simulink model "controller_2013B"  (R2013b)
settings: Solver=ode45  StartTime=0.0  StopTime=sim_time  FixedStep=0.001  RelTol=1e-3
InitFcn:
  | zh = 0.01;
undefined symbols (not defined in the file): Standard_Devices, UDP_Protocol, zh_step
libraries: rtwinlib x6, simulink x2, commutil2 x2, dspnetwork x2
settings Model: Creator=Lenka  LastModifiedBy=Anony
settings DebuggingCC: UnderspecifiedInitializationDetection=Simplified  MergeDetectMultiDrivingBlocksExec=error  FrameProcessingCompatibilityMsg=error
settings GRTTargetCC: CodeReplacementLibrary=C89/C90 (ANSI)

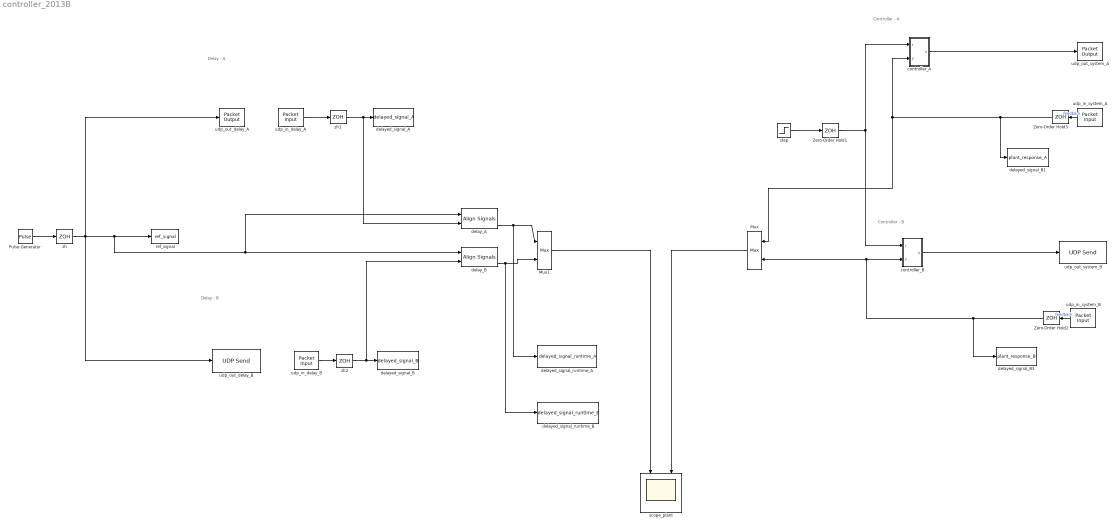
== system controller_2013B ==
  note: Controller - B
  note: Controller - A
  note: Delay - A
  note: Delay - B
  Mux : Mux  Inputs=2
  Mux1 : Mux  Inputs=2
  Pulse Generator : DiscretePulseGenerator  PulseType=Time based  Period=0.5  PulseWidth=0.1
  Zero-Order Hold1 : ZeroOrderHold  SampleTime=zh_step
  Zero-Order Hold2 : ZeroOrderHold  SampleTime=zh_step
  Zero-Order Hold3 : ZeroOrderHold  SampleTime=zh_step
  controller_A : Subsystem
  controller_B : Subsystem
  delay_A : commutil2/Align Signals  corrLength=800  stopUpdate=off  numConstDelay=3
  delay_B : commutil2/Align Signals  corrLength=800  stopUpdate=off  numConstDelay=3
  delayed_signal_A : ToWorkspace  VariableName=delayed_signal_A  SampleTime=zh_step  SaveFormat=Timeseries
  delayed_signal_B : ToWorkspace  VariableName=delayed_signal_B  SampleTime=zh_step  SaveFormat=Timeseries
  delayed_signal_B1 : ToWorkspace  VariableName=plant_response_A  SampleTime=zh_step  SaveFormat=Timeseries
  delayed_signal_B3 : ToWorkspace  VariableName=plant_response_B  SampleTime=zh_step  SaveFormat=Timeseries
  delayed_signal_runtime_A : ToWorkspace  VariableName=delayed_signal_runtime_A  SampleTime=zh_step  SaveFormat=Timeseries
  delayed_signal_runtime_B : ToWorkspace  VariableName=delayed_signal_runtime_B  SampleTime=zh_step  SaveFormat=Timeseries
  ref_signal : ToWorkspace  VariableName=ref_signal  SampleTime=zh_step  SaveFormat=Timeseries
  scope_plant : Scope  NumInputPorts=2
      settings: ShowLegends=on  YMin=0~0  YMax=325~1.3
  step : Step  SampleTime=0
  udp_in_delay_A : rtwinlib/Packet Input  SampleTime=0.001  MaxMissedTicks=inf  ShowMissedTicks=off  YieldWhenWaiting=off  DrvName=Standard_Devices/UDP_Protocol  DrvAddress=28000  DrvOptions=[2468394757 28000]  PacketSize=8  DataTypes='double'  ShowReady=off  ShowError=off  PacketID=1  ByteOrder=1  ShowTimestamp=off
      settings: AttributesFormatString=Standard Devices\nUDP Protocol [6978h]
  udp_in_delay_B : rtwinlib/Packet Input  SampleTime=0.001  MaxMissedTicks=inf  ShowMissedTicks=off  YieldWhenWaiting=off  DrvName=Standard_Devices/UDP_Protocol  DrvAddress=28010  DrvOptions=[2468394757 28010]  PacketSize=8  DataTypes='double'  ShowReady=off  ShowError=off  PacketID=1  ByteOrder=1  ShowTimestamp=off
      settings: AttributesFormatString=Standard Devices\nUDP Protocol [6982h]
  udp_in_system_A : rtwinlib/Packet Input  SampleTime=0.001  MaxMissedTicks=inf  ShowMissedTicks=off  YieldWhenWaiting=off  DrvName=Standard_Devices/UDP_Protocol  DrvAddress=28500  DrvOptions=[2468394757 28500]  PacketSize=8  DataTypes='double'  ShowReady=off  ShowError=off  PacketID=1  ByteOrder=1  ShowTimestamp=off
      settings: AttributesFormatString=Standard Devices\nUDP Protocol [6F54h]
  udp_in_system_B : rtwinlib/Packet Input  SampleTime=0.001  MaxMissedTicks=inf  ShowMissedTicks=off  YieldWhenWaiting=off  DrvName=Standard_Devices/UDP_Protocol  DrvAddress=28510  DrvOptions=[2468394757 28510]  PacketSize=8  DataTypes='double'  ShowReady=off  ShowError=off  PacketID=1  ByteOrder=1  ShowTimestamp=off
      settings: AttributesFormatString=Standard Devices\nUDP Protocol [6F54h]
  udp_out_delay_A : rtwinlib/Packet Output  SampleTime=0.01  MaxMissedTicks=inf  ShowMissedTicks=off  YieldWhenWaiting=off  DrvName=Standard_Devices/UDP_Protocol  DrvAddress=27000  DrvOptions=[2468394757 27000]  PacketSize=8  DataTypes='double'  ShowReady=off  ShowError=off  PacketID=1  ByteOrder=1  InitialValue=[]  FinalValue=[]
      settings: AttributesFormatString=Standard Devices\nUDP Protocol [6D60h]
  udp_out_delay_B : dspnetwork/UDP Send  remoteURL='147.32.183.5'  remotePort=27010  localURL='0.0.0.0'  localPortSource=Automatically determine  localPort=27000  sampletime=-1  separateLengthPort=0
  udp_out_system_A : rtwinlib/Packet Output  SampleTime=0.01  MaxMissedTicks=inf  ShowMissedTicks=off  YieldWhenWaiting=off  DrvName=Standard_Devices/UDP_Protocol  DrvAddress=27500  DrvOptions=[2468394757 27500]  PacketSize=8  DataTypes='double'  ShowReady=off  ShowError=off  PacketID=1  ByteOrder=1  InitialValue=[]  FinalValue=[]
      settings: AttributesFormatString=Standard Devices\nUDP Protocol [6B6Ch]
  udp_out_system_B : dspnetwork/UDP Send  remoteURL='147.32.183.5'  remotePort=27510  localURL='0.0.0.0'  localPortSource=Automatically determine  localPort=27000  sampletime=-1  separateLengthPort=0
  zh : ZeroOrderHold  SampleTime=zh_step
  zh1 : ZeroOrderHold  SampleTime=zh_step
  zh2 : ZeroOrderHold  SampleTime=zh_step
  wires:
  udp_in_system_A/1 -> Zero-Order Hold3/1  "feedback"
  step/1 -> Zero-Order Hold1/1
  controller_A/1(u) -> udp_out_system_A/1
  udp_in_system_B/1 -> Zero-Order Hold2/1  "feedback"
  controller_B/1(u) -> udp_out_system_B/1
  Mux/1 -> scope_plant/2
  Zero-Order Hold1/1 -> controller_A/1(r), controller_B/1(r)
  udp_in_delay_A/1 -> zh1/1
  zh1/1 -> delay_A/2, delayed_signal_A/1
  Pulse Generator/1 -> zh/1
  udp_in_delay_B/1 -> zh2/1
  zh2/1 -> delay_B/2, delayed_signal_B/1
  Mux1/1 -> scope_plant/1
  delay_B/3 -> delayed_signal_runtime_B/1, Mux1/2
  delay_A/3 -> delayed_signal_runtime_A/1, Mux1/1
  zh/1 -> udp_out_delay_A/1, udp_out_delay_B/1, delay_A/1, delay_B/1, ref_signal/1
  Zero-Order Hold2/1 -> delayed_signal_B3/1, controller_B/2(y), Mux/2
  Zero-Order Hold3/1 -> delayed_signal_B1/1, controller_A/2(y), Mux/1

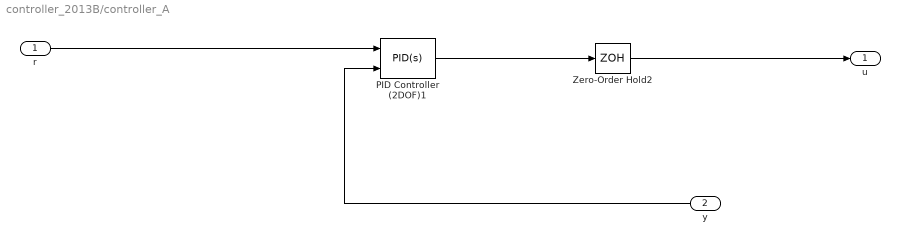
== system controller_2013B/controller_A ==
  r : Inport
  y : Inport  Port=2
  PID Controller (2DOF)1 : simulink/Continuous/PID Controller (2DOF)  Controller=PID  TimeDomain=Continuous-time  SampleTime=-1  IntegratorMethod=Forward Euler  FilterMethod=Forward Euler  Form=Parallel  P=6.3799380872686  I=2.12979603411331  D=3.6093223618413  N=48.5068620404972  b=2.39624043732871  c=0.716079145801974  InitialConditionSource=internal  InitialConditionForIntegrator=0  InitialConditionForFilter=0  ExternalReset=none  LimitOutput=off  UpperSaturationLimit=inf  LowerSaturationLimit=-inf  LinearizeAsGain=on  AntiWindupMode=none  Kb=1  TrackingMode=off  Kt=1  PParamMin=[]  PParamMax=[]  IParamMin=[]  IParamMax=[]  DParamMin=[]  DParamMax=[]  NParamMin=[]  NParamMax=[]  bParamMin=[]  bParamMax=[]  cParamMin=[]  cParamMax=[]  KbParamMin=[]  KbParamMax=[]  KtParamMin=[]  KtParamMax=[]  POutMin=[]  POutMax=[]  IOutMin=[]  IOutMax=[]  DOutMin=[]  DOutMax=[]  NOutMin=[]  NOutMax=[]  bOutMin=[]  bOutMax=[]  cOutMin=[]  cOutMax=[]  KbOutMin=[]  KbOutMax=[]  KtOutMin=[]  KtOutMax=[]  IntegratorOutMin=[]  IntegratorOutMax=[]  FilterOutMin=[]  FilterOutMax=[]  SumOutMin=[]  SumOutMax=[]  Sum1OutMin=[]  Sum1OutMax=[]  Sum2OutMin=[]  Sum2OutMax=[]  Sum3OutMin=[]  Sum3OutMax=[]  SumI1OutMin=[]  SumI1OutMax=[]  SumI2OutMin=[]  SumI2OutMax=[]  SumI3OutMin=[]  SumI3OutMax=[]  SumDOutMin=[]  SumDOutMax=[]  SaturationOutMin=[]  SaturationOutMax=[]  IntegratorContinuousStateAttributes=''  IntegratorStateMustResolveToSignalObject=off  IntegratorRTWStateStorageClass=Auto  FilterContinuousStateAttributes=''  FilterStateMustResolveToSignalObject=off  FilterRTWStateStorageClass=Auto
  Zero-Order Hold2 : ZeroOrderHold  SampleTime=zh_step
  u : Outport
  wires:
  r/1 -> PID Controller (2DOF)1/1
  y/1 -> PID Controller (2DOF)1/2
  Zero-Order Hold2/1 -> u/1
  PID Controller (2DOF)1/1 -> Zero-Order Hold2/1

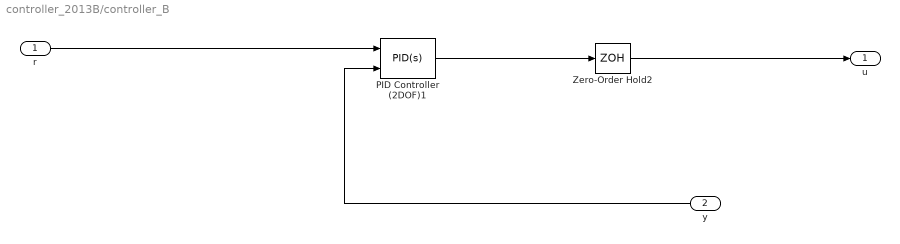
== system controller_2013B/controller_B ==
  r : Inport
  y : Inport  Port=2
  PID Controller (2DOF)1 : simulink/Continuous/PID Controller (2DOF)  Controller=PID  TimeDomain=Continuous-time  SampleTime=-1  IntegratorMethod=Forward Euler  FilterMethod=Forward Euler  Form=Parallel  P=6.3799380872686  I=2.12979603411331  D=3.6093223618413  N=48.5068620404972  b=2.39624043732871  c=0.716079145801974  InitialConditionSource=internal  InitialConditionForIntegrator=0  InitialConditionForFilter=0  ExternalReset=none  LimitOutput=off  UpperSaturationLimit=inf  LowerSaturationLimit=-inf  LinearizeAsGain=on  AntiWindupMode=none  Kb=1  TrackingMode=off  Kt=1  PParamMin=[]  PParamMax=[]  IParamMin=[]  IParamMax=[]  DParamMin=[]  DParamMax=[]  NParamMin=[]  NParamMax=[]  bParamMin=[]  bParamMax=[]  cParamMin=[]  cParamMax=[]  KbParamMin=[]  KbParamMax=[]  KtParamMin=[]  KtParamMax=[]  POutMin=[]  POutMax=[]  IOutMin=[]  IOutMax=[]  DOutMin=[]  DOutMax=[]  NOutMin=[]  NOutMax=[]  bOutMin=[]  bOutMax=[]  cOutMin=[]  cOutMax=[]  KbOutMin=[]  KbOutMax=[]  KtOutMin=[]  KtOutMax=[]  IntegratorOutMin=[]  IntegratorOutMax=[]  FilterOutMin=[]  FilterOutMax=[]  SumOutMin=[]  SumOutMax=[]  Sum1OutMin=[]  Sum1OutMax=[]  Sum2OutMin=[]  Sum2OutMax=[]  Sum3OutMin=[]  Sum3OutMax=[]  SumI1OutMin=[]  SumI1OutMax=[]  SumI2OutMin=[]  SumI2OutMax=[]  SumI3OutMin=[]  SumI3OutMax=[]  SumDOutMin=[]  SumDOutMax=[]  SaturationOutMin=[]  SaturationOutMax=[]  IntegratorContinuousStateAttributes=''  IntegratorStateMustResolveToSignalObject=off  IntegratorRTWStateStorageClass=Auto  FilterContinuousStateAttributes=''  FilterStateMustResolveToSignalObject=off  FilterRTWStateStorageClass=Auto
  Zero-Order Hold2 : ZeroOrderHold  SampleTime=zh_step
  u : Outport
  wires:
  PID Controller (2DOF)1/1 -> Zero-Order Hold2/1
  Zero-Order Hold2/1 -> u/1
  y/1 -> PID Controller (2DOF)1/2
  r/1 -> PID Controller (2DOF)1/1
